simulink model "last_pressed_led_detectchange"  (R2025a)
settings: Solver=FixedStepDiscrete  StartTime=0.0  StopTime=10  FixedStep=1  RelTol=1e-3
libraries: simulink x2
settings Model: Creator=mahij  LastModifiedBy=mahij

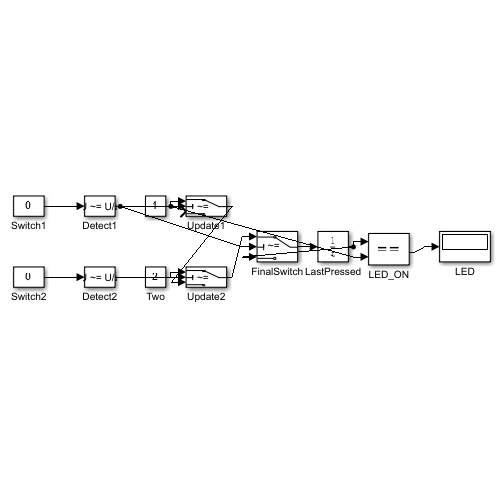
[thumbnail: Simulink's stored preview of the top-level diagram]
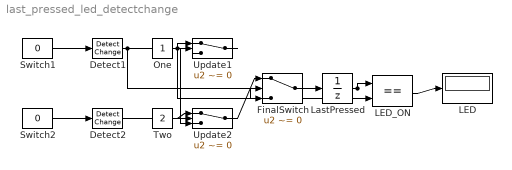
== system last_pressed_led_detectchange ==
  Detect1 : simulink/Logic and Bit Operations/Detect Change  vinit=0  OutDataTypeStr=boolean
  Detect2 : simulink/Logic and Bit Operations/Detect Change  vinit=0  OutDataTypeStr=boolean
  FinalSwitch : Switch  Criteria=u2 ~= 0  Threshold=0.5  SaturateOnIntegerOverflow=off  InputSameDT=off
  LED : Display
  LED_ON : RelationalOperator  Operator===  OutDataTypeStr=boolean  RndMeth=Simplest  InputSameDT=off
  LastPressed : UnitDelay  HasFrameUpgradeWarning=on
  One : Constant
  Switch1 : Constant  Value=0
  Switch2 : Constant  Value=0
  Two : Constant  Value=2
  Update1 : Switch  Criteria=u2 ~= 0  Threshold=0.5  SaturateOnIntegerOverflow=off  InputSameDT=off
  Update2 : Switch  Criteria=u2 ~= 0  Threshold=0.5  SaturateOnIntegerOverflow=off  InputSameDT=off
  wires:
  Switch1/1 -> Detect1/1
  Switch2/1 -> Detect2/1
  One/1 -> Update1/1, LED_ON/2
  Detect1/1 -> Update1/2, FinalSwitch/2
  Two/1 -> Update2/1
  Detect2/1 -> Update2/2
  Update1/1 -> Update2/3
  Update2/1 -> FinalSwitch/1
  LastPressed/1 -> FinalSwitch/3, LED_ON/1
  FinalSwitch/1 -> LastPressed/1
  LED_ON/1 -> LED/1
